simulink model "Cordova_Hydro_Diesel_ESS"  (R2020b)
settings: Solver=VariableStepAuto  StartTime=0.0  StopTime=8761  RelTol=1e-3
settings Model: Creator=jkarenzi  LastModifiedBy=michelechamberlin

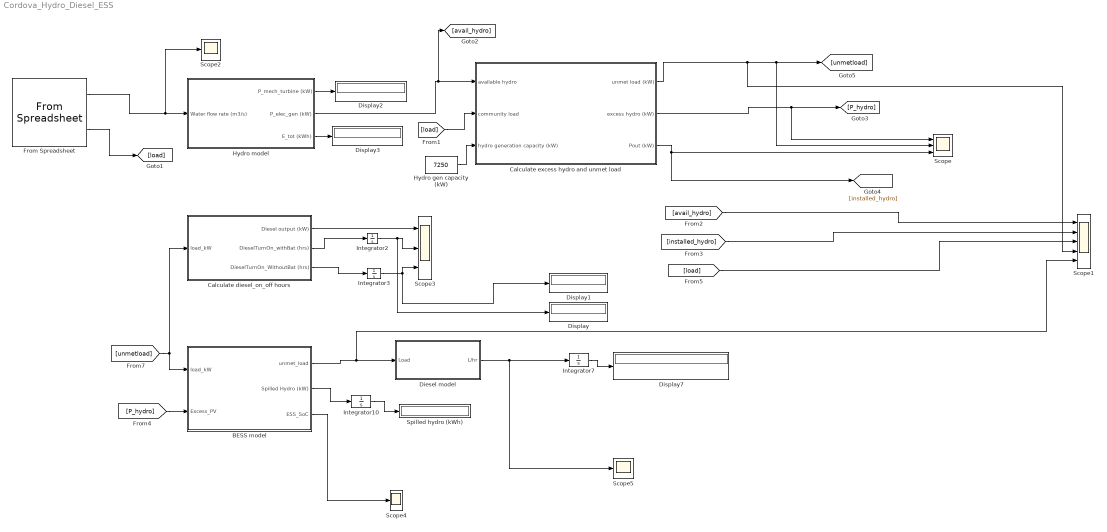
== system Cordova_Hydro_Diesel_ESS ==
  BESS model : Subsystem  TreatAsAtomicUnit=on  mask{P1=1000000, P2=100, P3=30, P4=90, P5=80}
      mask prompts: P1 "ESS Capacity"; P2 "Initial_SoC (%)"; P3 "Min_SoC (%)"; P4 "Max_SoC (%)"; P5 "Battery Efficieny (%)"
      mask init:
      | Bat_capacity = P1;
      | Init_SoC = P2;
      | min_SoC = P3;
      | max_SoC = P4;
      | bat_eff = P5;
  Calculate diesel_on_off hours : Subsystem  TreatAsAtomicUnit=on  mask{P1=1000, P2=0, P3=30, P4=90, P5=80}
      mask prompts: P1 "ESS Capacity"; P2 "Initial_SoC (%)"; P3 "Min_SoC (%)"; P4 "Max_SoC (%)"; P5 "Battery Efficieny (%)"
      mask init:
      | Bat_capacity = P1;
      | Init_SoC = P2;
      | min_SoC = P3;
      | max_SoC = P4;
      | bat_eff = P5;
  "Calculate excess hydro and unmet load " : Subsystem
  Diesel model : Subsystem  mask{P1=6000, P2=30, P3=820, P4=42.6, P5=960.58, P6=487.4}
      mask prompts: P1 "Diesel capacity (kW)"; P2 "Minimal loading point (%)"; P3 "density (kg/m3)"; P4 "LHV (MJ/kg)"; P5 "Fuel consumption at full load (L/hr)"; P6 "Fuel consumption at half load (L/hr)"
      mask init:
      | cap_kW = P1;
      | MLP = P2; %MLP: Minimal Loading Point
      | density = P3;
      | LHV = P4;
      | FL = P5;
      | HL = P6;
  Display{,1..3,7} (5 alike) : Display
  From Spreadsheet : FromSpreadsheet  FileName=C:\Users\michelechamberlin\Desktop\MicroFEWs\MATLAB Simulink\Cordova\Cordova.xlsx  SheetName=Sheet4  Range=A1:C8761  SampleTime=1
  Hydro gen capacity (kW) : Constant  Value=7250
  Hydro model : Subsystem  mask{P4=90, P5=10, P6=75}
      mask prompts: P4 "Available Head (m)"; P5 "Head loss (%)"; P6 "Turbine/Generator eff (%)"
      mask init:
      | h = P4;
      | h_loss = P5;
      | n = P6;
      mask DialogControl ParameterGroupVar Prompt: System details
  Integrator{2..3,7,10} (4 alike) : Integrator
  Scope : Scope  NumInputPorts=3
  Scope1 : Scope  NumInputPorts=5
  Scope2 : Scope
  Scope3 : Scope  NumInputPorts=3
  Scope4 : Scope
  Scope5 : Scope
  Spilled hydro (kWh) : Display
  wires:
  Calculate diesel_on_off hours/2(DieselTurnOn_withBat (hrs)) -> Integrator2/1
  Calculate diesel_on_off hours/3(DieselTurnOn_WithoutBat (hrs)) -> Integrator3/1
  Hydro model/1(P_mech_turbine (kW)) -> Display2/1
  Hydro model/3(E_tot (kWh)) -> Display3/1
  Diesel model/1(L/hr) -> Scope5/1, Integrator7/1
  Integrator7/1 -> Display7/1
  [P_hydro] -> BESS model/2(Excess_PV)
  BESS model/1(unmet_load) -> Scope1/5, Diesel model/1(Load)
  BESS model/2(Spilled Hydro (kW)) -> Integrator10/1
  Integrator10/1 -> Spilled hydro (kWh)/1
  BESS model/3(ESS_SoC) -> Scope4/1
  [unmetload] -> BESS model/1(load_kW), Calculate diesel_on_off hours/1(load_kW)
  Calculate diesel_on_off hours/1(Diesel output (kW)) -> Scope3/1
  Integrator3/1 -> Scope3/3, Display1/1
  [load] -> "Calculate excess hydro and unmet load "/2(community load)
  "Calculate excess hydro and unmet load "/1(unmet load (kW)) -> Scope1/4, Scope/2, [unmetload]
  "Calculate excess hydro and unmet load "/2(excess hydro (kW)) -> Scope/1, [P_hydro]
  Hydro gen capacity (kW)/1 -> "Calculate excess hydro and unmet load "/3(hydro generation capacity (kW))
  Hydro model/2(P_elec_gen (kW)) -> [avail_hydro], "Calculate excess hydro and unmet load "/1(available hydro)
  From Spreadsheet/1 -> Scope2/1, Hydro model/1(Water flow rate (m3/s))
  From Spreadsheet/2 -> [load]
  Integrator2/1 -> Display/1, Scope3/2
  "Calculate excess hydro and unmet load "/3(Pout (kW)) -> [installed_hydro], Scope/3
  [avail_hydro] -> Scope1/1
  [installed_hydro] -> Scope1/2
  [load] -> Scope1/3

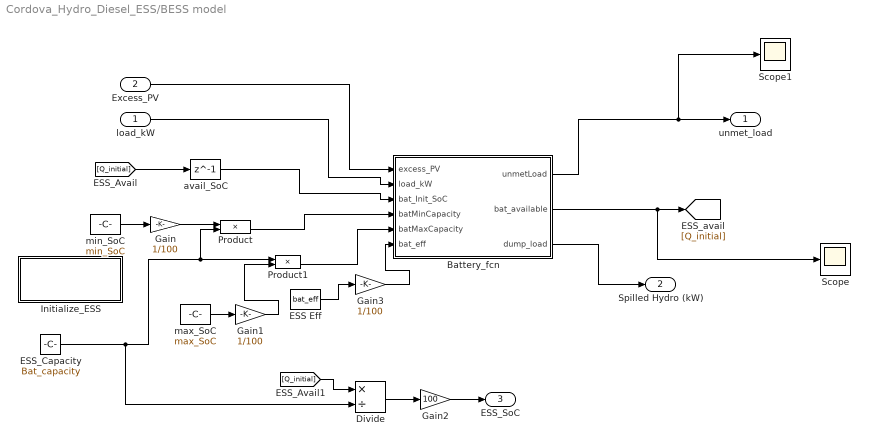
== system Cordova_Hydro_Diesel_ESS/BESS model ==
  load_kW : Inport
  Excess_PV : Inport  Port=2
  Battery_fcn : MATLAB Function  TreatAsAtomicUnit=on
  Divide : Product  Inputs=*/
  ESS Eff : Constant  Value=bat_eff
  "ESS_Capacity " : Constant  Value=Bat_capacity
  Gain : Gain  Gain=1/100
  Gain1 : Gain  Gain=1/100
  Gain2 : Gain  Gain=100
  Gain3 : Gain  Gain=1/100
  Initialize_ESS : Subsystem  TreatAsAtomicUnit=on
  Product : Product
  Product1 : Product
  Scope : Scope
  Scope1 : Scope
  avail_SoC : Delay  DelayLength=1  InitialCondition=0  SampleTime=1
  max_SoC : Constant  Value=max_SoC
  min_SoC : Constant  Value=min_SoC
  unmet_load : Outport
  Spilled Hydro (kW) : Outport  Port=2
  ESS_SoC : Outport  Port=3
  wires:
  Excess_PV/1 -> Battery_fcn/1(excess_PV)
  avail_SoC/1 -> Battery_fcn/3(bat_Init_SoC)
  Battery_fcn/1(unmetLoad) -> Scope1/1, unmet_load/1
  [Q_initial] -> avail_SoC/1
  max_SoC/1 -> Gain1/1
  min_SoC/1 -> Gain/1
  Gain/1 -> Product/1
  Product/1 -> Battery_fcn/4(batMinCapacity)
  Product1/1 -> Battery_fcn/5(batMaxCapacity)
  Gain1/1 -> Product1/2
  load_kW/1 -> Battery_fcn/2(load_kW)
  Battery_fcn/2(bat_available) -> Scope/1, [Q_initial]
  Battery_fcn/3(dump_load) -> Spilled Hydro (kW)/1
  ESS Eff/1 -> Gain3/1
  Gain3/1 -> Battery_fcn/6(bat_eff)
  "ESS_Capacity "/1 -> Divide/2, Product1/1, Product/2
  [Q_initial] -> Divide/1
  Divide/1 -> Gain2/1
  Gain2/1 -> ESS_SoC/1

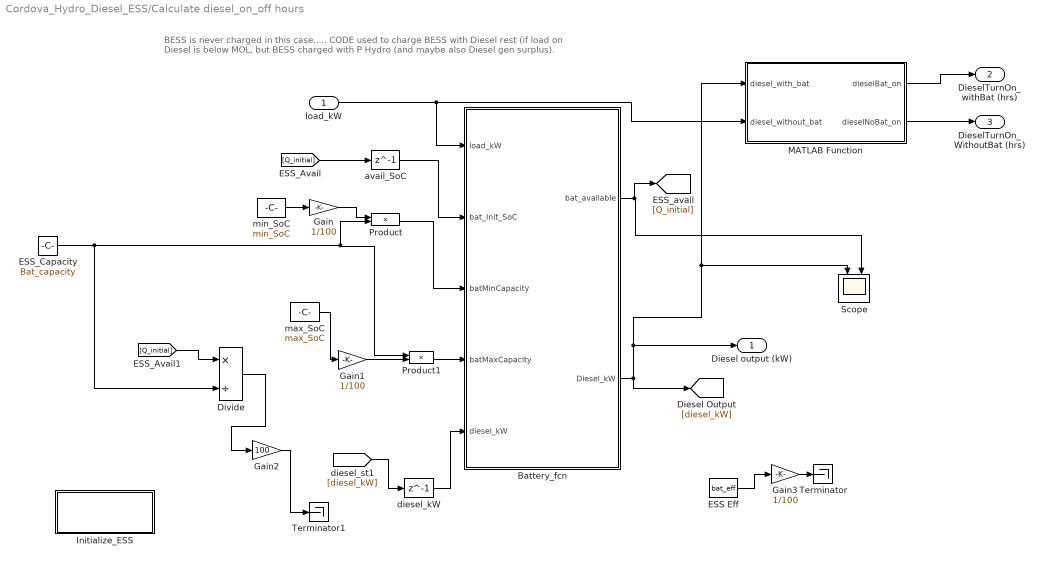
== system Cordova_Hydro_Diesel_ESS/Calculate diesel_on_off hours ==
  note: BESS is never charged in this case.....
      | CODE used to charge BESS with Diesel rest (if load on Diesel is below MOL, but BESS charged with P Hydro (and maybe also Diesel gen surplus).
  load_kW : Inport
  Battery_fcn : MATLAB Function  TreatAsAtomicUnit=on
  Divide : Product  Inputs=*/
  ESS Eff : Constant  Value=bat_eff
  "ESS_Capacity " : Constant  Value=Bat_capacity
  Gain : Gain  Gain=1/100
  Gain1 : Gain  Gain=1/100
  Gain2 : Gain  Gain=100
  Gain3 : Gain  Gain=1/100
  Initialize_ESS : Subsystem  TreatAsAtomicUnit=on
  MATLAB Function : MATLAB Function  TreatAsAtomicUnit=on
  Product : Product
  Product1 : Product
  Scope : Scope  NumInputPorts=2
  Terminator : Terminator
  Terminator1 : Terminator
  avail_SoC : Delay  DelayLength=1  InitialCondition=0  SampleTime=1
  diesel_kW : Delay  DelayLength=1  InitialCondition=0  SampleTime=1
  max_SoC : Constant  Value=max_SoC
  min_SoC : Constant  Value=min_SoC
  Diesel output (kW) : Outport
  DieselTurnOn_withBat (hrs) : Outport  Port=2
  DieselTurnOn_WithoutBat (hrs) : Outport  Port=3
  wires:
  Gain2/1 -> Terminator1/1
  Divide/1 -> Gain2/1
  [Q_initial] -> Divide/1
  "ESS_Capacity "/1 -> Product1/1, Product/2, Divide/2
  ESS Eff/1 -> Gain3/1
  Battery_fcn/2(Diesel_kW) -> [diesel_kW], Scope/1, MATLAB Function/1(diesel_with_bat), Diesel output (kW)/1
  Battery_fcn/1(bat_available) -> Scope/2, [Q_initial]
  load_kW/1 -> MATLAB Function/2(diesel_without_bat), Battery_fcn/1(load_kW)
  Gain1/1 -> Product1/2
  Product1/1 -> Battery_fcn/4(batMaxCapacity)
  Product/1 -> Battery_fcn/3(batMinCapacity)
  Gain/1 -> Product/1
  min_SoC/1 -> Gain/1
  max_SoC/1 -> Gain1/1
  [Q_initial] -> avail_SoC/1
  avail_SoC/1 -> Battery_fcn/2(bat_Init_SoC)
  Gain3/1 -> Terminator/1
  diesel_kW/1 -> Battery_fcn/5(diesel_kW)
  [diesel_kW] -> diesel_kW/1
  MATLAB Function/1(dieselBat_on) -> DieselTurnOn_withBat (hrs)/1
  MATLAB Function/2(dieselNoBat_on) -> DieselTurnOn_WithoutBat (hrs)/1

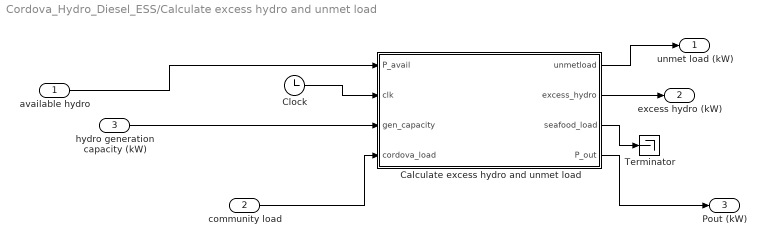
== system Cordova_Hydro_Diesel_ESS/Calculate excess hydro and unmet load  ==
  available hydro : Inport
  community load : Inport  Port=2
  hydro generation capacity (kW) : Inport  Port=3
  "Calculate excess hydro and unmet load " : MATLAB Function  TreatAsAtomicUnit=on
  Clock : Clock
  Terminator : Terminator
  unmet load (kW) : Outport
  excess hydro (kW) : Outport  Port=2
  Pout (kW) : Outport  Port=3
  wires:
  community load/1 -> "Calculate excess hydro and unmet load "/4(cordova_load)
  "Calculate excess hydro and unmet load "/1(unmetload) -> unmet load (kW)/1
  available hydro/1 -> "Calculate excess hydro and unmet load "/1(P_avail)
  "Calculate excess hydro and unmet load "/2(excess_hydro) -> excess hydro (kW)/1
  hydro generation capacity (kW)/1 -> "Calculate excess hydro and unmet load "/3(gen_capacity)
  Clock/1 -> "Calculate excess hydro and unmet load "/2(clk)
  "Calculate excess hydro and unmet load "/4(P_out) -> Pout (kW)/1
  "Calculate excess hydro and unmet load "/3(seafood_load) -> Terminator/1

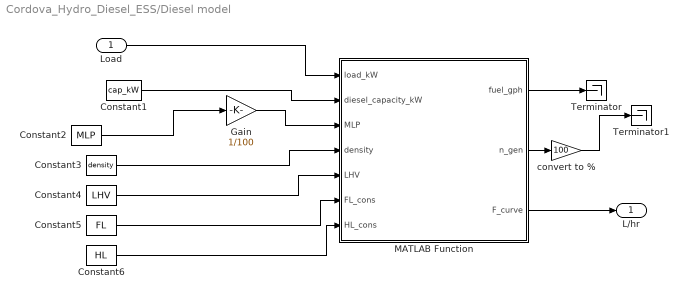
== system Cordova_Hydro_Diesel_ESS/Diesel model ==
  Load : Inport
  Constant1 : Constant  Value=cap_kW
  Constant2 : Constant  Value=MLP
  Constant3 : Constant  Value=density
  Constant4 : Constant  Value=LHV
  Constant5 : Constant  Value=FL
  Constant6 : Constant  Value=HL
  Gain : Gain  Gain=1/100
  MATLAB Function : MATLAB Function  TreatAsAtomicUnit=on
  Terminator : Terminator
  Terminator1 : Terminator
  convert to % : Gain  Gain=100
  L/hr : Outport
  wires:
  Load/1 -> MATLAB Function/1(load_kW)
  Constant1/1 -> MATLAB Function/2(diesel_capacity_kW)
  Constant2/1 -> Gain/1
  Gain/1 -> MATLAB Function/3(MLP)
  Constant3/1 -> MATLAB Function/4(density)
  Constant4/1 -> MATLAB Function/5(LHV)
  Constant5/1 -> MATLAB Function/6(FL_cons)
  Constant6/1 -> MATLAB Function/7(HL_cons)
  MATLAB Function/3(F_curve) -> L/hr/1
  MATLAB Function/2(n_gen) -> convert to %/1
  convert to %/1 -> Terminator1/1
  MATLAB Function/1(fuel_gph) -> Terminator/1

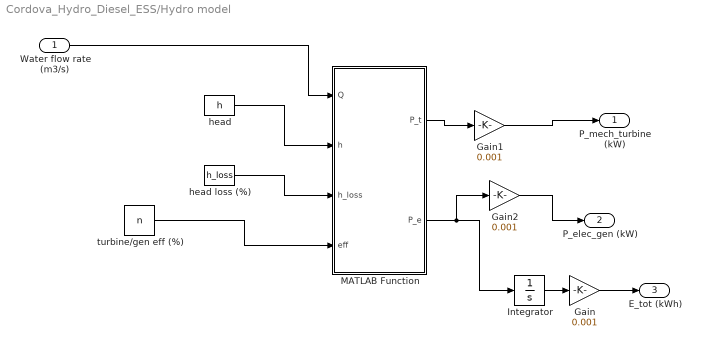
== system Cordova_Hydro_Diesel_ESS/Hydro model ==
  Water flow rate (m3/s) : Inport
  Gain : Gain  Gain=0.001
  Gain1 : Gain  Gain=0.001
  Gain2 : Gain  Gain=0.001
  Integrator : Integrator
  MATLAB Function : MATLAB Function  TreatAsAtomicUnit=on
  head : Constant  Value=h
  head loss (%) : Constant  Value=h_loss
  turbine/gen eff (%) : Constant  Value=n
  P_mech_turbine (kW) : Outport
  P_elec_gen (kW) : Outport  Port=2
  E_tot (kWh) : Outport  Port=3
  wires:
  Water flow rate (m3/s)/1 -> MATLAB Function/1(Q)
  head/1 -> MATLAB Function/2(h)
  MATLAB Function/2(P_e) -> Gain2/1, Integrator/1
  head loss (%)/1 -> MATLAB Function/3(h_loss)
  turbine/gen eff (%)/1 -> MATLAB Function/4(eff)
  Integrator/1 -> Gain/1
  Gain/1 -> E_tot (kWh)/1
  MATLAB Function/1(P_t) -> Gain1/1
  Gain1/1 -> P_mech_turbine (kW)/1
  Gain2/1 -> P_elec_gen (kW)/1

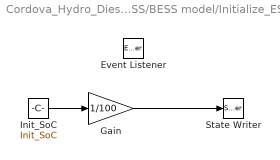
== system Cordova_Hydro_Diesel_ESS/BESS model/Initialize_ESS ==
  Event Listener : EventListener  DisableCoverage=on  EventName=reset
  Gain : Gain  Gain=1/100
  Init_SoC : Constant  Value=Init_SoC
  State Writer : StateWriter  StateOwnerBlock=../../avail_SoC
  wires:
  Init_SoC/1 -> Gain/1
  Gain/1 -> State Writer/1

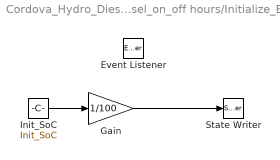
== system Cordova_Hydro_Diesel_ESS/Calculate diesel_on_off hours/Initialize_ESS ==
  Event Listener : EventListener  DisableCoverage=on  EventName=reset
  Gain : Gain  Gain=1/100
  Init_SoC : Constant  Value=Init_SoC
  State Writer : StateWriter  StateOwnerBlock=../../avail_SoC
  wires:
  Gain/1 -> State Writer/1
  Init_SoC/1 -> Gain/1

== matlab function Cordova_Hydro_Diesel_ESS/Calculate diesel_on_off hours/Battery_fcn ==
  data: load_kW input; bat_Init_SoC input; batMinCapacity input; batMaxCapacity input; bat_available output; Diesel_kW output; diesel_kW input
function [ bat_available,Diesel_kW] = batt_fcn(load_kW,bat_Init_SoC,batMinCapacity,batMaxCapacity,diesel_kW)
%Function to determine the impact of Cordova's 1 MW Battery 
%%%%%%%%%%%
%MJC: Not sure what the purpose of this function is, because it used to
%to be weird about BESS charging, but only output is BESS hours
%%%%%%%%%%

%initialize the bat_available, as well as the on/off status of the battery
%and diesel
bat_available = bat_Init_SoC;
% battery_st = Bat_st;
% Diesel_st = diesel_st;
Diesel_kW = diesel_kW; %MJC: from previous step (time delay block used 
min_loading_point = 400;  %minimal loading point of a 1MW diesel (40%)


%check if Bat can support available load
if(load_kW > 0 && load_kW <= (bat_available - batMinCapacity)) % MJC: BESS covers entire load
    
    bat_available = bat_available - load_kW
    Diesel_kW = 0
    
elseif (load_kW > 0 && load_kW > (bat_available - batMinCapacity)) % MJC: if BESS available, covers load. Diesel covers rest, or all
    
    bat_available = batMinCapacity;
    Diesel_kW = load_kW-(bat_available - batMinCapacity);
    % unmetLoad = 0; % Battery Picked up the load
    
    %If the load is greater than the batt cap., the gens should kick in
end


%if the unmet load is zero, diesel shouldn't kick in. bat SoC should remain
%same
if(load_kW==0)
    Diesel_kW=0;
end

%If battery drops to below 30%, diesel should kick in, pick up the load
%and charge the battery


if(bat_available < batMinCapacity)%MJC: With the changes implemented above, the model should never enter this stage
    fprintf(2,'Wrong Code somewhere, dude \n')
    if (( (load_kW + batMinCapacity) < min_loading_point) && (load_kW ~= 0))
        Diesel_kW = (min_loading_point) + (batMaxCapacity - batMinCapacity);
    else
        Diesel_kW = load_kW + (batMaxCapacity - batMinCapacity);
    end
    bat_available = batMaxCapacity;
    %     Bat_st = 0;
    
    %unmetLoad = load_kW;
end
end
 
 
 
 
 
% %Battery can't pick up the load, diesel should kick in and charge the
% %battery to 70% 
% if(diesel_st >0) 
%      if (( load_kW < min_loading_point) && (load_kW ~= 0))
%            Diesel_kW = (min_loading_point)* diesel_st; 
%            
%      else
%            Diesel_kW = load_kW * diesel_st; 
%      end
%  end
% 
% %If battery needs charging, diesel should kick in, pick up the load and 
% %full charge the battery
% if(Bat_st == 0) %battery needs charging
%           Diesel_kW = Diesel_kW + batMaxCapacity;
%           bat_available = batMaxCapacity;
% 
% end  
% end

== matlab function Cordova_Hydro_Diesel_ESS/Calculate diesel_on_off hours/MATLAB Function ==
  data: diesel_with_bat input; dieselBat_on output; diesel_without_bat input; dieselNoBat_on output
function [dieselBat_on,dieselNoBat_on] = fcn(diesel_with_bat,diesel_without_bat)
%MJC checked

if(diesel_with_bat<=0)
    dieselBat_on = 0;
else
    dieselBat_on = 1;
end

if(diesel_without_bat<=0)
    dieselNoBat_on = 0;
else
    dieselNoBat_on = 1;
end

== matlab function Cordova_Hydro_Diesel_ESS/Hydro model/MATLAB Function ==
  data: Q input; h input; h_loss input; P_t output; eff input; P_e output
function [P_t,P_e] = fcn(Q,h,h_loss,eff)
%h: dynamic head
%g: gravitational constant
%rho: density of water
h_dynamic = (1-(h_loss/100))*h;
h_dynamic = h_dynamic* 3.28; %convert to ft
Q = Q*15850.32; %convert to gpm
P_t = h_dynamic*Q/(5.30); %The eqn applies english units
P_e = P_t*(eff/100);

== matlab function Cordova_Hydro_Diesel_ESS/Calculate excess hydro and unmet load /Calculate excess hydro and unmet load  ==
  data: unmetload output; P_avail input; clk input; gen_capacity input; cordova_load input; excess_hydro output; seafood_load output; P_out output
function [unmetload,excess_hydro,seafood_load,P_out]  = fcn(P_avail,clk, gen_capacity,cordova_load)

P_out = P_avail;

%Calculate how PV is available and supply the load
avg_offseason_load = 3125; %average load in MW
%calcuate the added load due to the seafoods
T1 = 2881; %beginning of the fishing season
T2 = 6553; %End of the fishing season
%Estimate seafood loads
seafood_load = cordova_load - avg_offseason_load;
if(seafood_load <0)
    seafood_load = 0;
    
elseif(clk<T1)
    seafood_load = 0;
elseif(clk>T2)
    seafood_load = 0;
else
    %fprintf(2,'fishload')
    sprintf(2,clk)
    seafood_load = cordova_load - avg_offseason_load;
end



Cordova_non_seafood = cordova_load - seafood_load;


if(P_out > gen_capacity)
    P_out = gen_capacity;
end


if (P_out >= seafood_load)
   unemtLoad_seafood = 0;
   hydro_avail = P_out - seafood_load;
  
    else
       unemtLoad_seafood =  seafood_load- P_out;
       hydro_avail = 0;
end



if( hydro_avail > 0)
    if(hydro_avail  > Cordova_non_seafood)
        unemtLoad_cordova = 0;
    else
        unemtLoad_cordova = Cordova_non_seafood - hydro_avail;
    end
else
       unemtLoad_cordova =  Cordova_non_seafood;
end
   
excess_hydro = P_out - cordova_load; % due to capacity
excess_hydro_avail = P_avail - P_out; % due to the avail hydro  %% This does not make sense HERE, to me, but this variable is not used anywhere else....

if(excess_hydro<0)
    excess_hydro = 0;
end

unmetload = unemtLoad_cordova;

%Calculate how PV is available and supply the load
avg_offseason_load = 3125; %average load in MW
%calcuate the added load due to the seafoods
T1 = 2881; %beginning of the fishing season
T2 = 6553; %End of the fishing season

== matlab function Cordova_Hydro_Diesel_ESS/Diesel model/MATLAB Function ==
  data: load_kW input; fuel_gph output; diesel_capacity_kW input; MLP input; density input; LHV input; FL_cons input; HL_cons input; n_gen output; F_curve output
function [fuel_gph,n_gen,F_curve]  = fcn(load_kW,diesel_capacity_kW,MLP,density,LHV,FL_cons,HL_cons)
%MLP: minimum loading point
%LHV: Lower heating value
%FL_cons: fuel consumption at full load
%HL_consL fuel consumption at half load
slope = (FL_cons - HL_cons)/(diesel_capacity_kW - (diesel_capacity_kW/2));
%slope = 0.236;
intercept = HL_cons - (diesel_capacity_kW/2)*(slope);
%intercept = 0.72741;
F0 = intercept/diesel_capacity_kW;

n_gen = 3600*(load_kW/diesel_capacity_kW)/(density*(F0+slope*(load_kW/diesel_capacity_kW))*LHV);
%F_curve = F0*diesel_capacity + slope*(load_kW/diesel_capacity);



if(load_kW>diesel_capacity_kW)
    msg = 'Error: Available load greater than DEG capacity.';
    error(msg)
end
%specify the minimal laoding point of the diesel genset
min_load = MLP*diesel_capacity_kW; %MLP: Minimal loading point
if(load_kW<min_load)
    load_kW = min_load;
end
F_curve = F0*diesel_capacity_kW + slope.*load_kW;
A = 0.246; %L/kWh
B = 0.08415; %L/kWh
A_gal = 0.0650; %gal/kwh
B_gal = 0.02223; %gal/kwh 
fuel_gph = A_gal.*load_kW + B_gal.*diesel_capacity_kW; %eff in L/hr

== matlab function Cordova_Hydro_Diesel_ESS/BESS model/Battery_fcn ==
  data: excess_PV input; unmetLoad output; load_kW input; bat_Init_SoC input; batMinCapacity input; batMaxCapacity input; bat_eff input; bat_available output; dump_load output
function [ unmetLoad,bat_available,dump_load] = batt_fcn(excess_PV,load_kW,bat_Init_SoC,batMinCapacity,batMaxCapacity,bat_eff)
%if generation meets demand, no unmentload, energy storage unchanged, no
%excess renewable
%Here load_kW represents unmet load
bat_available = bat_Init_SoC;
%if load is greater than generation, use battery to cover the unmet load
if(load_kW > 0)
    %Check how much energy the battery has. If at minimum, send unmet
    %load to diesel
    if(bat_available<=batMinCapacity)
        bat_available = batMinCapacity;
        unmetLoad = load_kW;
        dump_load = 0 ;
        
        %If there's power in the battery, meet the load till the minimum is reached. then send
        %rest to the diesel
    elseif ((bat_available>batMinCapacity)&& (load_kW>(bat_available-batMinCapacity))) %batt avail greater bat min cap
        %  if(load_kW>(bat_available-batMinCapacity)) %unmet load > avail battery
        bat_available = batMinCapacity;
        unmetLoad = load_kW - (bat_Init_SoC - batMinCapacity);
        dump_load = 0 ;
        
    elseif((bat_available > batMinCapacity)&& (load_kW<=(bat_available-batMinCapacity)))
        
        bat_available = bat_Init_SoC - load_kW;
        unmetLoad = 0;
        dump_load = 0;
        
        %neglect self discharge rate
    else
        bat_available = bat_Init_SoC - load_kW;
        unmetLoad = 0;
        dump_load = 0 ;
    end
    % end
    %if generation meets demand and there's no excess PV
elseif ((load_kW == 0)&& (excess_PV ==0))
    bat_available =  bat_Init_SoC;
    unmetLoad = 0;
    dump_load = 0 ;
    %if there is excess PV, charge the ESS. Ignoring the self discharge rates
elseif(excess_PV >0)
    
    
    %  PVExcess = P_charge_kW - load_kW;
    if((bat_available+excess_PV/bat_eff)>=batMaxCapacity)
        dump_load = excess_PV-((batMaxCapacity-bat_available)/(bat_eff));%%MJC line was: dump_load = excess_PV
        bat_available = batMaxCapacity;
        unmetLoad = 0;
    else
        bat_available =  bat_available + excess_PV *(bat_eff);
        unmetLoad = 0;
        dump_load = 0;
    end
    
else
    bat_available = bat_Init_SoC;
    unmetLoad = 0;
    dump_load = 0;
end
end
